simulink library "carnot"  (R2013b)
settings: Solver=ode45  StartTime=0.0  StopTime=10.0  RelTol=1e-3
undefined symbols (not defined in the file or in its folder): A, acol, Ahabit, Awin, Azimuth_Angle, AziWin, B, C, c1, c4, capc, caph, CarnotCallbacks_Density, CarnotCallbacks_Enthalpy, CarnotCallbacks_Enthalpy2Temperature, CarnotCallbacks_Entropy, CarnotCallbacks_Evaporation_Enthalpy, CarnotCallbacks_GlobalMessageLevel, CarnotCallbacks_Grashof, CarnotCallbacks_Heat_Capacity, CarnotCallbacks_Kinematic_Viscosity, CarnotCallbacks_Prandtl, CarnotCallbacks_Saturation_Property, CarnotCallbacks_Saturation_Temperature, CarnotCallbacks_Saturation_Value_Water, CarnotCallbacks_Specific_Volume, CarnotCallbacks_Thermal_Conductivity, CarnotCallbacks_Vapour_Content, CarnotCallbacks_Vapour_Pressure, con, cond, d, Dd, density, dfin, dia, DiameterLastPiece, DPConstant, dpipe, DPLinear, DPQuadratic, emission_out, fluid, FluidMix, FluidType, FPC, frame, g, GeodeticHeight, Gwin, heat_capacity, hgt, HP, Hroom, ID, inlet, K, l, lin, lpipe ... (+29)
undefined symbols (not defined in the file): c2, c3, c5, c6, cwall, dactive, height, mc, mID, rho, tau, UAneighbour, UAwall, uloss
libraries: carnot x333, simulink x25, simulink_extras x7
(part 4 of 16)

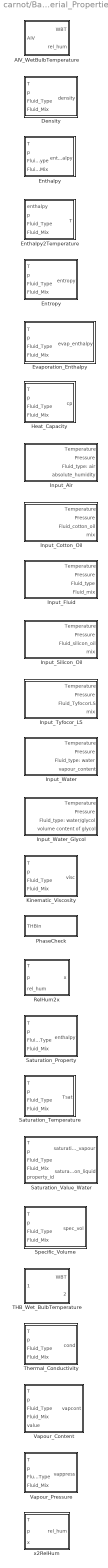
== system carnot/Basic/Material_Properties ==
  AIV_WetBulbTemperature : Subsystem  mask(AIV to wet bulb temperature and relative humidity){}
      mask help:
      | Calculate  - the relative humidity of air (rH)
      |                  - and the wet bulb temperature of air (WBT)
      | from          - dry bulb air temperature (DBT)
      |                  - and mass of water per mass of air (x)
      | in AIV vector.
      |
      | DBT        [degree centigrade]
      | p              [Pa]
      | x              kg water / kg air
      |
      | rel_hum   [percent]
      | WBT       [degree centigrade] -> T_WBT is valid for T [-6..40°C]
      mask Help: web(fullfile(path_carnot('help'),'wetbulbtemperature.html'),'-helpbrowser')
  Density : Subsystem  LoadFcn=CarnotCallbacks_Density('LoadFcn');  InitFcn=load('THB.mat');  VariantControl=CarlibClassic  mask(density){INPUTARGUMENTS=state variables (classic), DEBUGLEVEL=DEBUGLEVEL, MAXTOTALWARNINGS=inf, MAXCONSECUTIVEWARNINGS=inf, WRITETOFILE=0, FILENAME='errors.txt'}
      mask prompts: INPUTARGUMENTS "Input arguments"; DEBUGLEVEL "Debug level"; MAXTOTALWARNINGS "maximum number of total warning"; MAXCONSECUTIVEWARNINGS "maximum number of consecutive warnings"; WRITETOFILE "write messages to file"; FILENAME "filename for error messages"
      mask help:
      | Calculates the fluid density  [kg/m³]. Calls the function "density" in the CARNOT library "carlib".
      | You may use the block "GlobalMessageLevel" in the Toolbox to handle the debugging messages.
      | FluidType        Remarks
      | 1: water          fluid mix is vapourcontent in the 2-phase region
      | 2: air              fluid mix is (kg water) / (kg dry air)
      | 3: cotton oil       -
      | 4: silicone oil     -
      | 5: water-glycol   fluid mix is volume partition [0..1] of propylen glycol
      | 6: Tyfocor LS     function only available in liquid phase
      | 7: Water Constant = 998.21 kg/m³ (water at 20°C)
      | 8: Air Constant   = 1.118 kg/m³ (air at 20°C)
      mask init:
      | %Inports
      | CarnotCallbacks_Density('CreateInports');
      | 
      | %global debug level
      | [DEBUGLEVEL, MAXTOTALWARNINGS, MAXCONSECUTIVEWARNINGS, WRITETOFILE, FILENAME] = CarnotCallbacks_Density('CheckDebugLevels', DEBUGLEVEL, MAXTOTALWARNINGS, MAXCONSECUTIVEWARNINGS, WRITETOFILE, FILENAME);
      mask Help: web(fullfile(path_carnot('help'),'density.html'),'-helpbrowser')
      mask TypeOptions INPUTARGUMENTS: state variables (classic) | THB | THV
      mask Callback INPUTARGUMENTS: CarnotCallbacks_Density('MaskVisibilities');
      mask TypeOptions DEBUGLEVEL: DEBUGLEVEL | INFOLEVEL | WARNINGLEVEL | ERRORLEVEL | FATALLEVEL | NOLEVEL
  Enthalpy : Subsystem  LoadFcn=CarnotCallbacks_Enthalpy('LoadFcn');  InitFcn=load('THB.mat');  VariantControl=CarlibClassic  mask(enthalpy){INPUTARGUMENTS=state variables (classic), DEBUGLEVEL=WARNINGLEVEL, MAXTOTALMESSAGES=inf, MAXCONSECUTIVEMESSAGES=inf, WRITETOFILE=0, FILENAME='errors.txt'}
      mask prompts: INPUTARGUMENTS "Input arguments"; DEBUGLEVEL "Debug level"; MAXTOTALMESSAGES "maximum number of total warning"; MAXCONSECUTIVEMESSAGES "maximum number of consecutive warnings"; WRITETOFILE "write messages to file"; FILENAME "filename for error messages"
      mask help:
      | Calculates the fluid specific enthalpy  [J/kg].
      | Calls the CARNOT library "carlib".
      | WORKS FOR WATER AND DRY AIR! Enthalpy for other fluids is cp*T.
      | FluidType        Remarks
      | 1: water          fluid mix is vapourcontent in the 2-phase region
      | 2: air              fluid mix is (kg water) / (kg dry air)
      | 3: cotton oil       -
      | 4: silicone oil     -
      | 5: water-glycol   fluid mix is volume partition [0..1] of propylen glycol
      | 6: Tyfocor LS     function only available in liquid phase
      | 7: Water Constant = 0.0 J/kg (water at 20°C)
      | 8: Air Constant   = 0.0 J/kg (air at 20°C)
      mask init:
      | %Inports
      | CarnotCallbacks_Enthalpy('CreateInports');
      | 
      | %global debug level
      | [DEBUGLEVEL, MAXTOTALMESSAGES, MAXCONSECUTIVEMESSAGES, WRITETOFILE, FILENAME] = CarnotCallbacks_Enthalpy('CheckDebugLevels', DEBUGLEVEL, MAXTOTALMESSAGES, MAXCONSECUTIVEMESSAGES, WRITETOFILE, FILENAME);
      mask Help: web(fullfile(path_carnot('help'),'enthalpy.html'),'-helpbrowser')
      mask TypeOptions INPUTARGUMENTS: state variables (classic) | THB | THV
      mask Callback INPUTARGUMENTS: CarnotCallbacks_Enthalpy('MaskVisibilities');
      mask TypeOptions DEBUGLEVEL: DEBUGLEVEL | INFOLEVEL | WARNINGLEVEL | ERRORLEVEL | FATALLEVEL | NOLEVEL
  Enthalpy2Temperature : Subsystem  LoadFcn=CarnotCallbacks_Enthalpy2Temperature('LoadFcn');  VariantControl=CarlibClassic  mask(Enthalpy to Temperature){DEBUGLEVEL=WARNINGLEVEL, MAXTOTALMESSAGES=inf, MAXCONSECUTIVEMESSAGES=inf, WRITETOFILE=0, FILENAME='errors.txt'}
      mask prompts: DEBUGLEVEL "Debug level"; MAXTOTALMESSAGES "maximum number of total warning"; MAXCONSECUTIVEMESSAGES "maximum number of consecutive warnings"; WRITETOFILE "write messages to file"; FILENAME "filename for error messages"
      mask help:
      | Calculates the temperature  [°C] from the fluid Enthalpy [J/kg].
      | Enthalpy may be a scalar or a vector. All other inputs must be scalar.
      | FluidType        Remarks
      | 1: water          fluid mix is vapourcontent in the 2-phase region
      | 2: air              fluid mix is (kg water) / (kg dry air)
      | 3: cotton oil       -
      | 4: silicone oil     -
      | 5: water-glycol   fluid mix is volume partition [0..1] of propylen glycol
      | 6: Tyfocor LS     function only available in liquid phase
      | 7: Water Constant - function not defined
      | 8: Air Constant - function not defined
      mask init:
      | %global debug level
      | [DEBUGLEVEL, MAXTOTALMESSAGES, MAXCONSECUTIVEMESSAGES, WRITETOFILE, FILENAME] = CarnotCallbacks_Enthalpy2Temperature('CheckDebugLevels', DEBUGLEVEL, MAXTOTALMESSAGES, MAXCONSECUTIVEMESSAGES, WRITETOFILE, FILENAME);
      mask Help: web(fullfile(path_carnot('help'),'enthalpy2temperature.html'),'-helpbrowser')
      mask TypeOptions DEBUGLEVEL: DEBUGLEVEL | INFOLEVEL | WARNINGLEVEL | ERRORLEVEL | FATALLEVEL | NOLEVEL
      mask DialogControl ParameterTabVar0 Prompt: Debugging
  Entropy : Subsystem  LoadFcn=CarnotCallbacks_Entropy('LoadFcn');  InitFcn=load('THB.mat');  VariantControl=CarlibClassic  mask(entropy){INPUTARGUMENTS=state variables (classic), DEBUGLEVEL=WARNINGLEVEL, MAXTOTALMESSAGES=inf, MAXCONSECUTIVEMESSAGES=inf, WRITETOFILE=0, FILENAME='errors.txt'}
      mask prompts: INPUTARGUMENTS "Input arguments"; DEBUGLEVEL "Debug level"; MAXTOTALMESSAGES "maximum number of total warning"; MAXCONSECUTIVEMESSAGES "maximum number of consecutive warnings"; WRITETOFILE "write messages to file"; FILENAME "filename for error messages"
      mask help:
      | The block calculates the entropy  [J/kgK] of the fluid.
      | The block calls the function "entropy" in the CARNOT library "carlib".
      | FluidType        Remarks
      | 1: water          fluid mix is vapourcontent in the 2-phase region
      | 2: air              fluid mix is (kg water) / (kg dry air)
      | 3: cotton oil       -
      | 4: silicone oil     -
      | 5: water-glycol   fluid mix is volume partition [0..1] of propylen glycol
      | 6: Tyfocor LS     function only available in liquid phase
      | 7: Water Constant = 0.0 J/K/kg
      | 8: Air Constant   = 0.0 J/K/kg
      mask init:
      | %Inports
      | CarnotCallbacks_Entropy('CreateInports');
      | 
      | %global debug level
      | [DEBUGLEVEL, MAXTOTALMESSAGES, MAXCONSECUTIVEMESSAGES, WRITETOFILE, FILENAME] = CarnotCallbacks_Entropy('CheckDebugLevels', DEBUGLEVEL, MAXTOTALMESSAGES, MAXCONSECUTIVEMESSAGES, WRITETOFILE, FILENAME);
      mask Help: web(fullfile(path_carnot('help'),'entropy.html'),'-helpbrowser')
      mask TypeOptions INPUTARGUMENTS: state variables (classic) | THB | THV
      mask Callback INPUTARGUMENTS: CarnotCallbacks_Entropy('MaskVisibilities');
      mask TypeOptions DEBUGLEVEL: DEBUGLEVEL | INFOLEVEL | WARNINGLEVEL | ERRORLEVEL | FATALLEVEL | NOLEVEL
  Evaporation_Enthalpy : Subsystem  LoadFcn=CarnotCallbacks_Evaporation_Enthalpy('LoadFcn');  InitFcn=load('THB.mat');  VariantControl=CarlibClassic  mask(entropy){INPUTARGUMENTS=state variables (classic), DEBUGLEVEL=WARNINGLEVEL, MAXTOTALMESSAGES=inf, MAXCONSECUTIVEMESSAGES=inf, WRITETOFILE=0, FILENAME='errors.txt'}
      mask prompts: INPUTARGUMENTS "Input arguments"; DEBUGLEVEL "Debug level"; MAXTOTALMESSAGES "maximum number of total warning"; MAXCONSECUTIVEMESSAGES "maximum number of consecutive warnings"; WRITETOFILE "write messages to file"; FILENAME "filename for error messages"
      mask help:
      | The block calculates the evaporation enthalpy [J/kgK] of water.
      | The block uses the material properties functions in carlib.
      | FluidType  material           remarks on fluid mix
      | 1           water              vapourcontent in the 2-phase region
      | all others: function not defined
      mask init:
      | %Inports
      | CarnotCallbacks_Evaporation_Enthalpy('CreateInports');
      | 
      | %global debug level
      | [DEBUGLEVEL, MAXTOTALMESSAGES, MAXCONSECUTIVEMESSAGES, WRITETOFILE, FILENAME] = CarnotCallbacks_Evaporation_Enthalpy('CheckDebugLevels', DEBUGLEVEL, MAXTOTALMESSAGES, MAXCONSECUTIVEMESSAGES, WRITETOFILE, FILENAME);
      mask Help: web(fullfile(path_carnot('help'),'evaporation_enthalpy.html'),'-helpbrowser')
      mask TypeOptions INPUTARGUMENTS: state variables (classic) | THB | THV
      mask Callback INPUTARGUMENTS: CarnotCallbacks_Evaporation_Enthalpy('MaskVisibilities');
      mask TypeOptions DEBUGLEVEL: DEBUGLEVEL | INFOLEVEL | WARNINGLEVEL | ERRORLEVEL | FATALLEVEL | NOLEVEL
  Heat_Capacity : Subsystem  LoadFcn=CarnotCallbacks_Heat_Capacity('LoadFcn');  InitFcn=load('THB.mat');  VariantControl=CarlibClassic  mask(heat capacity){INPUTARGUMENTS=state variables (classic), DEBUGLEVEL=DEBUGLEVEL, MAXTOTALWARNINGS=inf, MAXCONSECUTIVEWARNINGS=inf, WRITETOFILE=0, FILENAME='errors.txt'}
      mask prompts: INPUTARGUMENTS "Input arguments"; DEBUGLEVEL "Debug level"; MAXTOTALWARNINGS "maximum number of total warning"; MAXCONSECUTIVEWARNINGS "maximum number of consecutive warnings"; WRITETOFILE "write messages to file"; FILENAME "filename for error messages"
      mask help:
      | Calculates the  heat_capacity of fluids [J/(kg*K)]. Calls calls the function "heat_capacity" in the CARNOT library "carlib".
      | You may use the block "GlobalMessageLevel" in the Toolbox to handle the debugging messages.
      | FluidType        Remarks
      | 1: water          fluid mix is vapourcontent in the 2-phase region
      | 2: air              fluid mix is (kg water) / (kg dry air)
      | 3: cotton oil       -
      | 4: silicone oil     -
      | 5: water-glycol   fluid mix is volume partition [0..1] of propylen glycol
      | 6: Tyfocor LS     function only available in liquid phase
      | 7: Water Constant = 4181.0 J/kg/K (water at 20°C)
      | 8: Air Constant   = 1007.0 J/kg/K (air at 20°C)
      mask init:
      | %Inports
      | CarnotCallbacks_Heat_Capacity('CreateInports');
      | 
      | %global debug level
      | [DEBUGLEVEL, MAXTOTALWARNINGS, MAXCONSECUTIVEWARNINGS, WRITETOFILE, FILENAME] = CarnotCallbacks_Heat_Capacity('CheckDebugLevels', DEBUGLEVEL, MAXTOTALWARNINGS, MAXCONSECUTIVEWARNINGS, WRITETOFILE, FILENAME);
      mask Help: web(fullfile(path_carnot('help'),'heat_capacity.html'),'-helpbrowser')
      mask TypeOptions INPUTARGUMENTS: state variables (classic) | THB | THV
      mask Callback INPUTARGUMENTS: CarnotCallbacks_Heat_Capacity('MaskVisibilities');
      mask TypeOptions DEBUGLEVEL: DEBUGLEVEL | INFOLEVEL | WARNINGLEVEL | ERRORLEVEL | FATALLEVEL | NOLEVEL
  Input_Air : Subsystem  mask(Input_Air){T=20, p=1e5, x=0.005}
      mask prompts: T "temperature (scalar or vector) [°C]"; p "pressure [Pa]"; x "absolute humidity of moist air [kg water/kg dry air]"
      mask help:
      | Input block for the material "Air"
      |
      | The relevant inputs for the calculation of the block can be specified as parameter in the mask
      mask Help: web(fullfile(path_carnot('help'),'input_material.html'),'-helpbrowser')
  Input_Cotton_Oil : Subsystem  mask(Input_Cotton_Oil){T=20, p=1e5}
      mask prompts: T "temperature (scalar or vector) [°C]"; p "pressure [Pa]"
      mask help: Input block for the material "Cotton Oil". The relevant inputs for the calculation of the block can be specified as parameter in the mask
      mask Help: web(fullfile(path_carnot('help'),'input_material.html'),'-helpbrowser')
  Input_Fluid : Subsystem  mask(Input_Fluid){fluid=Water, T=[10:10:50], p=1e5, x=0.005}
      mask prompts: fluid "Fluid type"; T "temperature (scalar or vector) [°C]"; p "pressure [Pa]"; x "Fluid Mix"
      mask help:
      | FLUID            FLUID MIX
      | water          vapourcontent in the 2-phase region
      | air               (kg water) / (kg dry air)
      | cotton oil       -
      | silicone oil     -
      | water-glycol   volume partition [0..1] of propylen glycol
      mask Help: web(fullfile(path_carnot('help'),'input_material.html'),'-helpbrowser')
      mask TypeOptions fluid: Water | Air | Cotton Oil | Silicone Oil | Water-Glycol Mix | Tyfocor LS | Water (Constant 20°C) | Air (dry+ constant 20°C)
  Input_Silicon_Oil : Subsystem  mask(Input_Silicon_Oil){T=20, p=1e5}
      mask prompts: T "temperature (scalar or vector) [°C]"; p "pressure [Pa]"
      mask help: Input block for the material "Silicon_Oil". The relevant inputs for the calculation of the block can be specified as parameter in the mask
      mask Help: web(fullfile(path_carnot('help'),'input_material.html'),'-helpbrowser')
  Input_Tyfocor_LS : Subsystem  mask(Input_Tyfocor_LS){T=20, p=1e5}
      mask prompts: T "temperature (scalar or vector) [°C]"; p "pressure [Pa]"
      mask help:
      | Input block for the material "Tyfocor_LS". The relevant inputs for the calculation of the block can be specified as parameter in the mask.
      | Tyfocor is a registered trademark of Tyforop Chemie, Hamburg (Germany).
      mask Help: web(fullfile(path_carnot('help'),'input_material.html'),'-helpbrowser')
  Input_Water : Subsystem  mask(Input_Water){T=20, p=2e6, xd=0}
      mask prompts: T "temperature (scalar or vector) [°C]"; p "pressure [Pa]"; xd "vapour content of the water [0..1]"
      mask help:
      | Input block for the material "Water"
      |
      | The relevant inputs for the calculation of the block can be specified as parameter in the mask
      mask Help: web(fullfile(path_carnot('help'),'input_material.html'),'-helpbrowser')
  Input_Water_Glycol : Subsystem  mask(input_water_glycol){T=20, p=1e5, g=0.4}
      mask prompts: T "temperature (scalar or vector) [°C]"; p "pressure [Pa]"; g "volume content of glycol [0..1]"
      mask help: Sets all values for the water - propylen-glycol mixtures.
      mask Help: web(fullfile(path_carnot('help'),'input_material.html'),'-helpbrowser')
  Kinematic_Viscosity : Subsystem  LoadFcn=CarnotCallbacks_Kinematic_Viscosity('LoadFcn');  InitFcn=load('THB.mat');  VariantControl=CarlibClassic  mask(kinematic viscosity){INPUTARGUMENTS=state variables (classic), DEBUGLEVEL=WARNINGLEVEL, MAXTOTALMESSAGES=inf, MAXCONSECUTIVEMESSAGES=inf, WRITETOFILE=0, FILENAME='errors.txt'}
      mask prompts: INPUTARGUMENTS "Input arguments"; DEBUGLEVEL "Debug level"; MAXTOTALMESSAGES "maximum number of total warning"; MAXCONSECUTIVEMESSAGES "maximum number of consecutive warnings"; WRITETOFILE "write messages to file"; FILENAME "filename for error messages"
      mask help:
      | Calculates the kinematic viscosity of fluids [m²/s].
      | Calls the function "viscosity" in the CARNOT library "carlib".
      | FluidType        Remarks
      | 1: water          fluid mix is vapourcontent in the 2-phase region
      | 2: air              fluid mix is (kg water) / (kg dry air)
      | 3: cotton oil       -
      | 4: silicone oil     -
      | 5: water-glycol   fluid mix is volume partition [0..1] of propylen glycol
      | 6: Tyfocor LS     function only available in liquid phase
      | 7: Water Constant = 1.004e-6 m²/s (water at 20°C)
      | 8: Air Constant   = 15.35e-6 m²/s (air at 20°C)
      mask init:
      | %Inports
      | CarnotCallbacks_Kinematic_Viscosity('CreateInports');
      | 
      | %global debug level
      | [DEBUGLEVEL, MAXTOTALMESSAGES, MAXCONSECUTIVEMESSAGES, WRITETOFILE, FILENAME] = CarnotCallbacks_Kinematic_Viscosity('CheckDebugLevels', DEBUGLEVEL, MAXTOTALMESSAGES, MAXCONSECUTIVEMESSAGES, WRITETOFILE, FILENAME);
      mask Help: web(fullfile(path_carnot('help'),'kinematic_viscosity.html'),'-helpbrowser')
      mask TypeOptions INPUTARGUMENTS: state variables (classic) | THB | THV
      mask Callback INPUTARGUMENTS: CarnotCallbacks_Kinematic_Viscosity('MaskVisibilities');
      mask TypeOptions DEBUGLEVEL: DEBUGLEVEL | INFOLEVEL | WARNINGLEVEL | ERRORLEVEL | FATALLEVEL | NOLEVEL
  PhaseCheck : Subsystem  mask(phasecheck){}
      mask help: Checks whether fluid is still in the correct phase, for example if water is not steam or ice. Simulation is stopped for inconstistent phase.
      mask Help: web(fullfile(path_carnot('help'),'phase_check.html'),'-helpbrowser')
  RelHum2x : Subsystem  mask(relative humidity to x){}
      mask help:
      | Calculate the mass of water per mass of air (x)
      | from the relative humidity of air.
      |
      | T             [degree centigrade]
      | p             [Pa]
      | rel_hum   [percent]
      | x              kg water / kg air
      mask Help: web(fullfile(path_carnot('help'),'rel_hum2x.html'),'-helpbrowser')
  Saturation_Property : Subsystem  LoadFcn=CarnotCallbacks_Saturation_Property('LoadFcn');  InitFcn=load('THB.mat');  VariantControl=CarlibClassic  mask(saturation property){INPUTARGUMENTS=state variables (classic), PROPERTY=density, FLUIDPHASE=liquid, DEBUGLEVEL=WARNINGLEVEL, MAXTOTALMESSAGES=inf, MAXCONSECUTIVEMESSAGES=inf, WRITETOFILE=0, FILENAME='errors.txt'}
      mask prompts: INPUTARGUMENTS "Input arguments"; FLUIDPHASE "fluid phase"; DEBUGLEVEL "Debug level"; MAXTOTALMESSAGES "maximum number of total warning"; MAXCONSECUTIVEMESSAGES "maximum number of consecutive warnings"; WRITETOFILE "write messages to file"; FILENAME "filename for error messages"
      mask help:
      | The block calculates the saturation value of water by the value of a specified property. Calls the function "saturationproperty" in the CARNOT library "Carlib".
      |
      | PROPERTY            UNIT
      | density                     kg/m³
      | heat capacity           J/kgK
      | heat conductivity     W/mK
      | kinematic viscosity   m²/s
      | enthalpy                   J/kg
      | entropy                     J/kgK
      | prandtl                      --
      | specific volume        m³/kg
      mask init:
      | %Inports
      | CarnotCallbacks_Saturation_Property('CreateInports');
      | 
      | %global debug level
      | [DEBUGLEVEL, MAXTOTALMESSAGES, MAXCONSECUTIVEMESSAGES, WRITETOFILE, FILENAME] = CarnotCallbacks_Saturation_Property('CheckDebugLevels', DEBUGLEVEL, MAXTOTALMESSAGES, MAXCONSECUTIVEMESSAGES, WRITETOFILE, FILENAME);
      mask Help: web(fullfile(path_carnot('help'),'saturationproperty.html'),'-helpbrowser')
      mask TypeOptions INPUTARGUMENTS: state variables (classic) | THB | THV
      mask Callback INPUTARGUMENTS: CarnotCallbacks_Saturation_Property('MaskVisibilities');
      mask TypeOptions PROPERTY: density | heat capacity | heat conductivity | kinematic viscosity | enthalpy | entropy | prandtl | specific volume
      mask TypeOptions FLUIDPHASE: vaporous | liquid | solid
      mask TypeOptions DEBUGLEVEL: DEBUGLEVEL | INFOLEVEL | WARNINGLEVEL | ERRORLEVEL | FATALLEVEL | NOLEVEL
  Saturation_Temperature : Subsystem  LoadFcn=CarnotCallbacks_Saturation_Temperature('LoadFcn');  InitFcn=load('THB.mat');  VariantControl=CarlibClassic  mask(Saturation Temperature){INPUTARGUMENTS=state variables (classic), DEBUGLEVEL=WARNINGLEVEL, MAXTOTALMESSAGES=inf, MAXCONSECUTIVEMESSAGES=inf, WRITETOFILE=0, FILENAME='errors.txt'}
      mask prompts: INPUTARGUMENTS "Input arguments"; DEBUGLEVEL "Debug level"; MAXTOTALMESSAGES "maximum number of total warning"; MAXCONSECUTIVEMESSAGES "maximum number of consecutive warnings"; WRITETOFILE "write messages to file"; FILENAME "filename for error messages"
      mask help:
      | Calculates the saturationtemperature in °C
      | Fluid Type 1 - water or water mixtures: temperature of saturated steam as a function of pressure.
      | Fluid Type 2 - moist air: dew point temperature of the moist air as a function of water content. Input fluid mix (kg water / kg air) may be a vector.
      mask init:
      | %Inports
      | CarnotCallbacks_Saturation_Temperature('CreateInports');
      | 
      | %global debug level
      | [DEBUGLEVEL, MAXTOTALMESSAGES, MAXCONSECUTIVEMESSAGES, WRITETOFILE, FILENAME] = CarnotCallbacks_Saturation_Temperature('CheckDebugLevels', DEBUGLEVEL, MAXTOTALMESSAGES, MAXCONSECUTIVEMESSAGES, WRITETOFILE, FILENAME);
      mask Help: web(fullfile(path_carnot('help'),'saturation_temperature.html'),'-helpbrowser')
      mask TypeOptions INPUTARGUMENTS: state variables (classic) | THB | THV
      mask Callback INPUTARGUMENTS: CarnotCallbacks_Saturation_Temperature('MaskVisibilities');
      mask TypeOptions DEBUGLEVEL: DEBUGLEVEL | INFOLEVEL | WARNINGLEVEL | ERRORLEVEL | FATALLEVEL | NOLEVEL
  Saturation_Value_Water : Subsystem  LoadFcn=CarnotCallbacks_Saturation_Value_Water('LoadFcn');  InitFcn=load('THB.mat');  VariantControl=CarlibClassic  mask(saturation value water){INPUTARGUMENTS=state variables (classic), DEBUGLEVEL=WARNINGLEVEL, MAXTOTALMESSAGES=inf, MAXCONSECUTIVEMESSAGES=inf, WRITETOFILE=0, FILENAME='errors.txt'}
      mask prompts: INPUTARGUMENTS "Input arguments"; DEBUGLEVEL "Debug level"; MAXTOTALMESSAGES "maximum number of total warning"; MAXCONSECUTIVEMESSAGES "maximum number of consecutive warnings"; WRITETOFILE "write messages to file"; FILENAME "filename for error messages"
      mask help:
      | Calculates the saturation value of fluid by the value of a specified property.
      | Temperature may be a scalar or vector, all other inputs must be scalar.
      | property-ID        property                       unit
      | 1                       density                         [kg/m³]
      | 2                       heat capacity               [J/kgK]
      | 3                       heat conductivity         [W/mK]
      | 4                       kinematic viscosity       [m²/s]
      | 5                       enthalpy                       [J/kg]
      | 6                       entropy                         [J/kgK]
      | 7                       prandtl                          [-]
      | 8                       specific volume            [m³/kg]
      | not defined for this function
      | 9                       evaporation  enthalpy  [J/kg]
      | 10                     vapourpressure            [Pa]
      | 11                     saturationtemperatur    [°C]
      mask init:
      | %Inports
      | CarnotCallbacks_Saturation_Value_Water('CreateInports');
      | 
      | %global debug level
      | [DEBUGLEVEL, MAXTOTALMESSAGES, MAXCONSECUTIVEMESSAGES, WRITETOFILE, FILENAME] = CarnotCallbacks_Saturation_Value_Water('CheckDebugLevels', DEBUGLEVEL, MAXTOTALMESSAGES, MAXCONSECUTIVEMESSAGES, WRITETOFILE, FILENAME);
      mask Help: web(fullfile(path_carnot('help'),'saturationvalue_water.html'),'-helpbrowser')
      mask TypeOptions INPUTARGUMENTS: state variables (classic) | THB | THV
      mask Callback INPUTARGUMENTS: CarnotCallbacks_Saturation_Value_Water('MaskVisibilities');
      mask TypeOptions DEBUGLEVEL: DEBUGLEVEL | INFOLEVEL | WARNINGLEVEL | ERRORLEVEL | FATALLEVEL | NOLEVEL
  Specific_Volume : Subsystem  LoadFcn=CarnotCallbacks_Specific_Volume('LoadFcn');  InitFcn=load('THB.mat');  VariantControl=CarlibClassic  mask(specific volume){INPUTARGUMENTS=state variables (classic), DEBUGLEVEL=DEBUGLEVEL, MAXTOTALWARNINGS=inf, MAXCONSECUTIVEWARNINGS=inf, WRITETOFILE=0, FILENAME='errors.txt'}
      mask prompts: INPUTARGUMENTS "Input arguments"; DEBUGLEVEL "Debug level"; MAXTOTALWARNINGS "maximum number of total warning"; MAXCONSECUTIVEWARNINGS "maximum number of consecutive warnings"; WRITETOFILE "write messages to file"; FILENAME "filename for error messages"
      mask help:
      | Calculates the specific volume of fluids [m³/kg]. Calls the function "specific_volume" in the CARNOT library "Carlib".
      | You may use the block "GlobalMessageLevel" in the Toolbox to handle the debugging messages.
      | FluidType        Remarks
      | 1: water          fluid mix is vapourcontent in the 2-phase region
      | 2: air              fluid mix is (kg water) / (kg dry air)
      | 3: cotton oil       -
      | 4: silicone oil     -
      | 5: water-glycol   fluid mix is volume partition [0..1] of propylen glycol
      | 6: Tyfocor LS     function only available in liquid phase
      | 7: Water Constant = 1.0 / 998.21 m³/kg (water at 20°C)
      | 8: Air Constant   = 1.0 / 1.118 m³/kg (air at 20°C)
      mask init:
      | %Inports
      | CarnotCallbacks_Specific_Volume('CreateInports');
      | 
      | %global debug level
      | [DEBUGLEVEL, MAXTOTALWARNINGS, MAXCONSECUTIVEWARNINGS, WRITETOFILE, FILENAME] = CarnotCallbacks_Specific_Volume('CheckDebugLevels', DEBUGLEVEL, MAXTOTALWARNINGS, MAXCONSECUTIVEWARNINGS, WRITETOFILE, FILENAME);
      mask Help: web(fullfile(path_carnot('help'),'specific_volume.html'),'-helpbrowser')
      mask TypeOptions INPUTARGUMENTS: state variables (classic) | THB | THV
      mask Callback INPUTARGUMENTS: CarnotCallbacks_Specific_Volume('MaskVisibilities');
      mask TypeOptions DEBUGLEVEL: DEBUGLEVEL | INFOLEVEL | WARNINGLEVEL | ERRORLEVEL | FATALLEVEL | NOLEVEL
  THB_Wet_BulbTemperature : Subsystem  mask(THB to wet bulb temperature and relative humidity){}
      mask help:
      | Calculate  - the relative humidity of air (rH)
      |                  - and the wet bulb temperature of air (WBT)
      | from          - dry bulb air temperature (DBT)
      |                  - and mass of water per mass of air (x)
      | in THV vector.
      |
      | DBT        [degree centigrade]
      | p              [Pa]
      | x              kg water / kg air
      |
      | rel_hum   [percent]
      | WBT       [degree centigrade] -> T_WBT is valid for T [-6..40°C]
      mask Help: web(fullfile(path_carnot('help'),'wetbulbtemperature.html'),'-helpbrowser')
  Thermal_Conductivity : Subsystem  LoadFcn=CarnotCallbacks_Thermal_Conductivity('LoadFcn');  InitFcn=load('THB.mat');  VariantControl=CarlibClassic  mask(thermal conductivity){INPUTARGUMENTS=state variables (classic), DEBUGLEVEL=WARNINGLEVEL, MAXTOTALMESSAGES=inf, MAXCONSECUTIVEMESSAGES=inf, WRITETOFILE=0, FILENAME='errors.txt'}
      mask prompts: INPUTARGUMENTS "Input arguments"; DEBUGLEVEL "Debug level"; MAXTOTALMESSAGES "maximum number of total warning"; MAXCONSECUTIVEMESSAGES "maximum number of consecutive warnings"; WRITETOFILE "write messages to file"; FILENAME "filename for error messages"
      mask help:
      | Calclulates the heat conductivity of fluids in [W/(m*K)]. Calls the function "cond" in the CARNOT library "carlib".
      | Temperature input may be a vector with several elements.
      | You may use the block "GlobalMessageLevel" in the Toolbox to handle the debugging messages.
      | FluidType        Remarks
      | 1: water          fluid mix is vapourcontent in the 2-phase region
      | 2: air              fluid mix is (kg water) / (kg dry air)
      | 3: cotton oil       -
      | 4: silicone oil     -
      | 5: water-glycol   fluid mix is volume partition [0..1] of propylen glycol
      | 6: Tyfocor LS     function only available in liquid phase
      | 7: Water Constant =  0.5984 W/m/K (water at 20°C)
      | 8: Air Constant   =  0.02569 W/m/K (air at 20°C)
      mask init:
      | %Inports
      | CarnotCallbacks_Thermal_Conductivity('CreateInports');
      | 
      | %global debug level
      | [DEBUGLEVEL, MAXTOTALMESSAGES, MAXCONSECUTIVEMESSAGES, WRITETOFILE, FILENAME] = CarnotCallbacks_Thermal_Conductivity('CheckDebugLevels', DEBUGLEVEL, MAXTOTALMESSAGES, MAXCONSECUTIVEMESSAGES, WRITETOFILE, FILENAME);
      mask Help: web(fullfile(path_carnot('help'),'thermal_conductivity.html'),'-helpbrowser')
      mask TypeOptions INPUTARGUMENTS: state variables (classic) | THB | THV
      mask Callback INPUTARGUMENTS: CarnotCallbacks_Thermal_Conductivity('MaskVisibilities');
      mask TypeOptions DEBUGLEVEL: DEBUGLEVEL | INFOLEVEL | WARNINGLEVEL | ERRORLEVEL | FATALLEVEL | NOLEVEL
  Vapour_Content : Subsystem  LoadFcn=CarnotCallbacks_Vapour_Content('LoadFcn');  InitFcn=load('THB.mat');  VariantControl=CarlibClassic  mask(vapourcontent){INPUTARGUMENTS=state variables (classic), PROPERTYTYPE=density, DEBUGLEVEL=WARNINGLEVEL, MAXTOTALMESSAGES=inf, MAXCONSECUTIVEMESSAGES=inf, WRITETOFILE=0, FILENAME='errors.txt'}
      mask prompts: INPUTARGUMENTS "Input arguments"; PROPERTYTYPE "property type"; DEBUGLEVEL "Debug level"; MAXTOTALMESSAGES "maximum number of total warning"; MAXCONSECUTIVEMESSAGES "maximum number of consecutive warnings"; WRITETOFILE "write messages to file"; FILENAME "filename for error messages"
      mask help:
      | The block calculates the (water-)vapour content of water or water-glycol mixture by the value of a specified property. The block calls the function "vapourcontent" in the CARNOT library "Carlib".
      | Temperature and the "Value" may be a scalar or vector, all other inputs must be scalar (length of "temperature" and "value" must be same).
      | You may use the block "GlobalMessageLevel" in the Toolbox to handle the debugging messages.
      | Definition of property-types
      | property                    unit
      |  density                     [kg/m³]
      |  heat capacity           [J/kgK]
      |  heat conductivity     [W/mK]
      |  kinematic viscosity   [m²/s]
      |  enthalpy                   [J/kg]
      |  entropy                     [J/kgK]
      |  prandtl                      [-]
      |  specific volume        [m³/kg]
      mask init:
      | %Inports
      | CarnotCallbacks_Vapour_Content('CreateInports');
      | 
      | %global debug level
      | [DEBUGLEVEL, MAXTOTALMESSAGES, MAXCONSECUTIVEMESSAGES, WRITETOFILE, FILENAME] = CarnotCallbacks_Vapour_Content('CheckDebugLevels', DEBUGLEVEL, MAXTOTALMESSAGES, MAXCONSECUTIVEMESSAGES, WRITETOFILE, FILENAME);
      mask Help: web(fullfile(path_carnot('help'),'vapour_content.html'),'-helpbrowser')
      mask TypeOptions INPUTARGUMENTS: state variables (classic) | THB | THV
      mask Callback INPUTARGUMENTS: CarnotCallbacks_Vapour_Content('MaskVisibilities');
      mask TypeOptions PROPERTYTYPE: density | heat capacity | heat conductivity | kinematic viscosity | enthalpy | entropy | prandtl | specific volume
      mask TypeOptions DEBUGLEVEL: DEBUGLEVEL | INFOLEVEL | WARNINGLEVEL | ERRORLEVEL | FATALLEVEL | NOLEVEL
  Vapour_Pressure : Subsystem  LoadFcn=CarnotCallbacks_Vapour_Pressure('LoadFcn');  InitFcn=load('THB.mat');  VariantControl=CarlibClassic  mask(vapourpressure){INPUTARGUMENTS=state variables (classic), DEBUGLEVEL=WARNINGLEVEL, MAXTOTALMESSAGES=inf, MAXCONSECUTIVEMESSAGES=inf, WRITETOFILE=0, FILENAME='errors.txt'}
      mask prompts: INPUTARGUMENTS "Input arguments"; DEBUGLEVEL "Debug level"; MAXTOTALMESSAGES "maximum number of total warning"; MAXCONSECUTIVEMESSAGES "maximum number of consecutive warnings"; WRITETOFILE "write messages to file"; FILENAME "filename for error messages"
      mask help:
      | Calculates the vapour pressure of fluids [Pa]. Calls the function "vapourpressure" in the CARNOT library "Carlib".
      | You may use the block "GlobalMessageLevel" in the Toolbox to handle the debugging messages.
      | FluidType        Remarks
      | 1: water          fluid mix is vapourcontent in the 2-phase region
      | 2: air              fluid mix is (kg water) / (kg dry air)
      | 3: cotton oil       function not defined
      | 4: silicone oil     function not defined
      | 5: water-glycol   fluid mix is volume partition [0..1] of propylen glycol
      | 6: Tyfocor LS     function only available in liquid phase
      | 7: Water Constant function not defined
      | 8: Air Constant   function not defined
      mask init:
      | %Inports
      | CarnotCallbacks_Vapour_Pressure('CreateInports');
      | 
      | %global debug level
      | [DEBUGLEVEL, MAXTOTALMESSAGES, MAXCONSECUTIVEMESSAGES, WRITETOFILE, FILENAME] = CarnotCallbacks_Vapour_Pressure('CheckDebugLevels', DEBUGLEVEL, MAXTOTALMESSAGES, MAXCONSECUTIVEMESSAGES, WRITETOFILE, FILENAME);
      mask Help: web(fullfile(path_carnot('help'),'vapourpressure.html'),'-helpbrowser')
      mask TypeOptions INPUTARGUMENTS: state variables (classic) | THB | THV
      mask Callback INPUTARGUMENTS: CarnotCallbacks_Vapour_Pressure('MaskVisibilities');
      mask TypeOptions DEBUGLEVEL: DEBUGLEVEL | INFOLEVEL | WARNINGLEVEL | ERRORLEVEL | FATALLEVEL | NOLEVEL
  x2RelHum : Subsystem  mask(x to relative humidity){}
      mask help:
      | Calculate  the relative humidity of air
      | from the mass of water per mass of air (x).
      |
      | T             [°C]
      | p             [Pa]
      | rel_hum   [percent]
      | x              kg water / kg dry air
      mask Help: web(fullfile(path_carnot('help'),'x2rel_hum.html'),'-helpbrowser')

== system carnot/Basic/Pressure_Drop ==
  Pressure_Drop_Collector : Subsystem  mask(Pressure Drop Collector){len=1, lin=10, qua=10}
      mask prompts: len "Length of Collector"; lin "lin: linear pressure drop in Pa/(kg/s)"; qua "qua: quadratic pressure drop in Pa/(kg/s)²"
      mask help:
      | Calculates the pressure drop according to constant values of con, lin and qua:
      | dp_dyn = con + lin*mdot + qua*mdot²
      | Static height is taken in account via the collector inclination, the length and the temperatures:
      | dp_stat = density * grav * height
      | Total pressure is dp = dp_dyn + dpstat
      mask Help: web(fullfile(path_carnot('help'),'Pressure_Drop_Collector.html'),'-helpbrowser')
  Pressure_Drop_Fix : Subsystem  mask(fixed pressure drop){con=con, lin=lin, qua=qua}
      mask prompts: con "c : constant (static) pressure drop in Pa"; lin "l : linear pressure drop Pa/(kg/s)"; qua "q : quadratic pressure drop Pa/(kg/s)²"
      mask help:
      | Constant parameters for pressure drop in a flow.
      | dp = c + l*mdot + q*mdot²
      | Calculation is done for ID > 10000 (dp = f(l, q), c is neglected) and ID > 20000 (dp = f(c,l,q)).
      | Applied directly to the THB bus.
      mask Help: web(fullfile(path_carnot('help'),'Pressure_Drop_Fix.html'),'-helpbrowser')
  Pressure_Drop_PipeTheory : Subsystem  mask(theoretical pressure drop of a pipe){dia=0.02, len=1, rough=0.04, nbend=1}
      mask prompts: dia "Diameter in m"; len "Length of pipe in m"; rough "Roughness of pipe in m"; nbend "Number of 90° bends"
      mask help: Calculates the pressure drop in a pipe according to a theoretical model.
      mask Help: web(fullfile(path_carnot('help'),'Pressure_Drop_PipeTheory.html'),'-helpbrowser')
  Pressure_Drop_StorageHX : Subsystem  mask(Pressure drop of tube heat exchanger in a storage){dia=dia, hgt=hgt}
      mask prompts: dia "Diameter in m"; hgt "height difference inlet-outlet"
      mask help:
      | Calculates the pressure drop in a tube heat exchanger according to:
      | dp = qua*mdot^2 + lin*mdot + density*grav*height
      mask Help: web(fullfile(path_carnot('help'),'Pressure_Drop_StorageHX.html'),'-helpbrowser')
  Pressure_Drop_StoragePipe : Subsystem  mask(Pressure drop pipe connection of a storage){dia=dia, hgt=hgt}
      mask prompts: dia "Diameter in m"; hgt "height difference inlet-outlet"
      mask help:
      | Calculates the pressure drop in a pipe connection to a storage according to:
      | dp = qua*mdot^2 + lin*mdot + density*grav*height
      | The temperature for the density is taken from the storage nodes.
      mask Help: web(fullfile(path_carnot('help'),'Pressure_Drop_StoragePipe.html'),'-helpbrowser')
  Pressure_Drop_changeD : Subsystem  mask(Pressure Drop Change Diameter){dia=dia}
      mask prompts: dia "Diameter in m"
      mask help: Calculates the pressure drop due to a diameter change at the inlet (of a pipe).
      mask Help: web(fullfile(path_carnot('help'),'Pressure_Drop_changeD.html'),'-helpbrowser')
  Pressure_Drop_staticHeight : Subsystem  mask(Pressure Drop static Height){}
      mask help:
      | Pressure drop or increase due to statig height.
      | Calculation is done for ID > 20000 (dp = f(h)).
      | dp = height/Nnodes*grav*density(Tnodes)
      | The length of Tnodes defines the number of temperature nodes.
      | The height is between inlet and outlet. It is divided by the number of nodes Nnodes in the temperature vector "Tnodes".
      | Height is positive for outlet above inlet but pressure decreases.
      mask Help: web(fullfile(path_carnot('help'),'Pressure_Drop_staticHeight.html'),'-helpbrowser')
  Pressuredrop : Subsystem  mask(pressure drop){}
      mask help:
      | Pressure drop according to input values of con, lin and qua:
      | dp = con + lin*mdot + qua*mdot²
      | The coefficients are also added to the correponding THB elements.
      mask Help: web(fullfile(path_carnot('help'),'Pressuredrop.html'),'-helpbrowser')

== system carnot/Basic/Thermal_Models ==
  Combustion_Calculation : Subsystem  TreatAsAtomicUnit=on
  HeatPump_basic : Subsystem  mask(heat pump){K=K, caph=caph, capc=capc, UA=UA}
      mask prompts: K "Parameters K (see also HP_param.m)"; caph "thermal capacity hot loop [J/K]"; capc "thermal capacity cold loop [J/K]"; UA "heat loss coefficient [W/K]"
      mask help:
      | Linearized heat pump model, uses measured data according to EN 14511 as input (Schwamberger, K.: Fortschrittsberichete VDI, Nr. 263, 1991).
      | heating power: Qdot_h = K1*Tcold_in + K2*Thot_out + K3
      | electric power: Pel = K4*Tcold_in + K5*Thot_out + K6
      | source power: Qdot_c = -K7*Tcold_in - K8*Thot_out - K9
      | differential equation: cap*dTh/dt = Qdot + mdot*cp*(T_in-T) + UA*(Tamb-T)
      | with: cap = mass * heat_capactiy
      | See hp_param.m for the parameters K1 to K9.
      mask Help: web(fullfile(path_carnot('help'),'HeatPump_basic.html'),'-helpbrowser')
      mask Display: plot(0,-30,120,130,[30,46,36,46,36,46,30],[40,40,50,60,70,80,80],[70,54,64,54,64,54,64,54,64,54,70],[40,40,44,50,55,60,65,70,75,80,80],[56,45],[95,95],[51,51],[82,95])
  House_OneNodeModel : Subsystem  mask(House One Node Model){Ahabit=Ahabit, Hroom=Hroom, tini=tini, UAout=UAwall, mc=mc, UAin=UAneighbour, dtroom=inf, AziWin=AziWin, Awin=Awin, Uwin=Uwin, Gwin=Gwin}
      mask prompts: Ahabit "living surface in m²"; Hroom "height of rooms in m"; tini "initial temperature"; UAout "heat loss of walls and roof in W/K"; mc "total thermal capacity in J/K"; UAin "heat transfer to neighbour in W/K"; dtroom "LIMITED TEMPERATURE CHANGE in K (standard value = 'inf')"; AziWin "orientation of 4 windows (south 0, east -90,west 90)"; Awin "surface of 4 windows in m² (vector)"; Uwin "heat loss coefficient 4 windows in W/m²/K [vector]"; Gwin "light transmittance 4 windows (0..1) * (1 - frame_part) [vector]"
      mask help:
      | Simple model of 1-node room or house. The differential equation is solved:
      | (m*c)house * dT/dt = solar_gain + internal_gain + heating_power - losses_to_ambient - losses_to_neighbour_room
      | The heating power is generated by a radiator or floor heating system. A usual value for the internal gains is 2.3 W/m².
      | The windows have a shading for solar radiation (standard value is 1):
      | solar gain = Solar_Radiation_on_window * light_transmittance * shading_factor
      | Use "look under mask" to set up the models parameters (initial conditions, surfaces characteristics...).
      |
      | LIMITED TEMPERATURE CHANGE: If you want to calculate idealized heating behaviour. 0 K means that the room temperature is fixed, the power balace is the theoretical heating demand (see example_House_Ideal.mdl).
      mask init:
      | invmc = 1/mc;
      | Gwin = max(0,min(1,Gwin));
      mask Help: web(fullfile(path_carnot('help'),'Simple_House.html'),'-helpbrowser')
      mask Display: plot(0,-15,80,100,[30,30,60,60,30],[20,50,50,20,20],[47,47,56,56,47],[40,30,30,40,40],[42,42,34,34],[20,40,40,20],[62,45,28],[48,70,48])
  Pipe_basic : Subsystem  mask(Pipe basic){vol=pi*(d/2)^2*l, L=l, uloss=uloss, effcond=cond, cwall=cwall, t0=t0, nodes=nodes}
      mask prompts: vol "Volume [m³]"; L "Length of pipe [m]"; uloss "Heat loss per pipe length [W/(m*K)]"; effcond "Effective conductivity of pipe wall [W/(m*K)]"; cwall "Capacity of pipewall per length [J/(m*K)]"; t0 "initial temperature [degree centigrade]"; nodes "number of nodes"
      mask help:
      | Multinode pipe with capacity. The flow is calculated by the upwind scheme heat conduction between nodes by central differences (Patankar 1980).
      | heat loss: u = conductivity / ( d_in * ln (d_out / d_in) )
      mask init:
      | nodes = max(nodes, 1);
      | vnode = max(vol,0.0001)/nodes;
      | lnode = max(L, 0.001)/nodes;
      | cnode = max(0.001,cwall)*L/vnode;
      | unode = uloss*lnode/vnode;
      | cond = effcond/(lnode*lnode);
      mask Help: web(fullfile(path_carnot('help'),'Pipe_basic.html'),'-helpbrowser')
      mask Display: plot(0,0,100,100,[24,27,27,24,75,80,80,75,24,20,20,24],[60,53,46,40,40,46,55,60,60,53,46,40])
  Radiator_basic : Subsystem  mask(basic Radiator){pnomEN=1000, dtnomEN=50, expo=1.5, mcp=10*4200}
      mask prompts: pnomEN "Qdot_nom: nominal power in W"; dtnomEN "Tdiff_nom: nominal temperature difference in K"; expo "radiator exponent (> 0)"; mcp "mass * capacity per unit in J/K"
      mask help:
      | The block calculates the heat transfer of a radiator to a room according to the EN 442 equation.
      | Qdot = Qdot_nom * (Tdiff/Tdiff_nom)^n
      mask init:
      | mcap = max(1,mcp); % lower limit for capacity is 1 J/K
      | 
      | % correct values because current model 
      | % uses outlet temperature as mean temperature
      | pnom = pnomEN;
      | dtnom = dtnomEN-5;
      mask Help: web(['file:///' fullfile(path_carnot('help'),'Radiator.html')],'-helpbrowser')
  Solar_Collector_basic : Subsystem  mask(Basic Solar Thermal Collector){acol=acol, c1=c1, c2=c2, c3=c3, c4=c4, c5=c5, c6=c6, tini=tini}
      mask prompts: acol "A : collector surface  [m²]"; c1 "c1 : heat loss coefficient at (Tm-Ta)=0  [W/(m²*K)]"; c2 "c2: temperature dependence of the heat loss coefficient [W/(m*K)²]"; c3 "c3 : wind speed dependence of the heat loss coefficient [J/(m³K)]"; c4 "c4 : sky temperature dependence of the heat loss coefficient [W/(m²K)]"; c5 "c5 : effective thermal capacity [J/(m²K)]"; c6 "c6 : wind dependence in the zero loss efficiency [s/m]"; tini "initial temperature [degree centigrade]"
      mask help: Model according to EN 12975 / ISO 22975
      mask Help: web(fullfile(path_carnot('help'),'Solar_Collector_basic.html'),'-helpbrowser')
      mask Display: disp('solar thermal\ncollector\nEN 12975')
  T_Ground_Undisturbed : Subsystem  mask(Undisturbed ground temperature){Tmeanoutside=0, deltathetae=10, tshift=0, cond_ground=1, rhocp=1000*2000, hh=10, znodes=10}
      mask prompts: Tmeanoutside "mean outside temperature over one year [°C]"; deltathetae "amplitude of monthly outside temperatures [°C]"; tshift "time shift where external temperature sine-curve shows a minimum [h]"; cond_ground "soil thermal conductivity in W/m/K"; rhocp "soil heat capacity per Volume in J/m³/K"; hh "depth z in m"; znodes "number of nodes"
      mask help:
      | The temperature of the undisturbed ground Tg is caclulated for a number of equidistant nodes from the surface down to a depth z.
      |
      | Tg = Tavg - dTavg * exp(-z/dg) * cos(2*pi*(t-ts)/t0 - z/dg) + G*z
      |
      | penetration depth : dg = sqrt(t0*cond/(pi*dens*cp))
      |
      | cond  : thermal conductivity of the ground in W/m/K
      | cp    : heat capacity of the ground in J/kg/K
      | dens  : density of the ground in kg/m³
      | G     : temperature increase in the depth (= 0.03 K/m)
      | t     : time of the year in seconds
      | t0    : total seconds of one year (= 3600*24*365)
      | ts    : time in seconds where the ambient temperature curve shows a minimum
      | Tavg  : annual mean ambient temperature
      | dTavg : annual amplitude of the ambient temperature
      | z     : depth in meters
      |
      | The equation is based on approaches presented in the literature for seasonal temperature variations in the earth’s crust (Baehr & Stephan 2006; Wesselak & Schabbach 2009), neglecting the influence of the heat transfer resistance from the ambient air to the surface of the ground (i.e. u_surf =):
      mask init:
      | %thermische eindringtiefe
      | delta_grd = sqrt((8760*3600*cond_ground)/(pi*rhocp));
      | 
      | % height vector
      | z = [0:hh/znodes:hh];
      mask Help: web(fullfile(path_carnot('help'),'T_Ground_Undisturbed.html'),'-helpbrowser')
      mask Display: plot(0,0,100,100,[90,10],[90,90],[50,50],[-0,90],[49,48,46,44,41,34,25,15],[-0,20,40,50,60,70,80,90],[52,54,56,58,61,67,76,85],[-0,20,40,50,60,70,80,90],[50,49,49,48,48,48,50,54,60],[-0,20,30,40,50,60,70,80,90],[50,51,51,52,52,50,48,43,35],[0,20,30,40,50,60,70,80,90])
  Thermal_Capacity : Subsystem  mask(Thermal Capacity){UA=1, mcp=4182*10, Tamb=20, cp_approx=4000}
      mask prompts: UA "Loss coefficient in W/K"; mcp "Thermal capacity in J/K"; Tamb "Ambient temperature in °C"; cp_approx "heat capacity of fluid in J/kg/K (approximate value)"
      mask help: Basic one node model of a thermal mass using the differential equation:
      mask Help: web(fullfile(path_carnot('help'),'Thermal_Capacity.html'),'-helpbrowser')
  Thermal_Node : Subsystem  mask(Thermal Capacity){UA=1, mcp=10*4182, cp_approx=4182, Tini=20}
      mask prompts: UA "Loss coefficient of node in W/K"; mcp "Thermal capacity of the node (mcp) in J/K"; cp_approx "Heat capacity of entering massflow in J/kg/K (approximate value)"; Tini "Initial temperature in °C"
      mask help:
      | Basic one node model of a thermal mass using the differential equation:
      | mcp * dT/dt = UA_loss*(Tamb-T) + mdot*cp_in*(Tin-T) + Qdot
      | Qdot: additional thermal power added to node
      | mdot: entering massflow
      | Tin: temperature of entering massflow
      mask Help: web(fullfile(path_carnot('help'),'Thermal_Capacity.html'),'-helpbrowser')
      mask Display: plot(-20,0,120,100,[10,70,70,10,10],[10,10,70,70,10],[70,90,90,30,10],[10,30,90,90,70],[90,70],[90,70],[50,30],[60,60],[40,40],[30,60])
  Wall_basic : Subsystem  mask(Wall basic){tau=tau, t0=t0, d=d, dactive=dactive, cond=cond, cwall=cwall, rho=rho}
      mask prompts: tau "Time constant in s"; t0 "Initial temperature in °C"; d "Thickness of layers in m"; dactive "Depth of active layer(s) in m"; cond "Conductivity of layer material in W/m/K"; cwall "Capacity of layer material in J/kg/K"; rho "Density of layer material in kg/m³"
      mask help: Basic model of a wall using a multilayer Beuken model.
      mask Help: web(fullfile(path_carnot('help'),'Wall_basic.html'),'-helpbrowser')
  sfun_storageTnodes : Subsystem  mask(S-Function Storage T-Nodes){dia=0.5, volume=0.5, standing=1, uloss=1.1, ubot=1.1, utop=1.1, cond=0.9, tini=20, nodes=10, nconnect=10}
      mask prompts: dia "diameter [m]"; volume "volume [m³]"; standing "standing cylinder"; uloss "heat transfer coefficient to ambient [W/m²K]"; ubot "heat transfer coefficient to ambient bottom [W/m²K]"; utop "heat transfer coefficient to ambient top [W/m²K]"; cond "effective thermal conductivity [W/mK]"; tini "initial temperature [°C]"; nodes "number of nodes [1]"; nconnect "number of ports [1]"
      mask help:
      | Basic 1xN Model for a storage tank based on the equation. The flow is calculated by the upwind scheme heat conduction between nodes by central differences (Patankar 1980).
      | (rho*cp) * dT/dt =U * Aloss / Vnode * (Tamb - Tnode)
      | + cond / dh2 * (Tnode_above - Tnode)
      | + cond / dh2 * (Tnode_below - Tnode)
      | + mdot_up * cp / Vnode * (Tnode_below - Tnode)
      | + mdot_down * cp / Vnode * (Tnode_above - Tnode)
      | + Uhx * Ahx / Vnode * (Thx_node - Tnode)
      mask init:
      | if (floor(nodes)-nodes>eps(nodes)) || nodes < 1.0
      |     error('The number of nodes must be a positve integer!');
      | end
      | 
      | if (floor(nconnect)-nconnect>eps(nconnect)) || nconnect < 1.0
      |     error('The number of ports must be a positve integer!');
      | end
      | 
      | 
      | 
      | if numel(tini)==1
      |     tini = ones(int32(nodes), 1)*tini;
      | else
      |     if numel(tini)~=int32(nodes)
      |         error('The initialisation temperature must be a scalar or a vector of size of number of nodes!');
      |     end
      | end
      | 
      | CarnotCallbacks_storage_Tnodes('InitCallback', gcb, nconnect);
      mask Help: web(fullfile(path_carnot('help'),'sfun_storageTnodes.html'),'-helpbrowser')
  sfun_storage_heatexchanger : Subsystem  mask(storage heat exchanger){idn=finned tube theoretical  - stratified, nodes=nodes, inlet=inlet, outlet=outlet, pp=[dpipe, swall, lpipe, cond, dfin, sfin, nfin]}
      mask prompts: idn "type"; nodes "number of nodes"; inlet "inlet node"; outlet "outlet node"; pp "parameter vector"
      mask init:
      | switch(idn)
      |     case 1
      |         id = 201;
      |     case 2
      |         id = 301;
      |     case 3
      |         id = 202;
      |     case 4
      |         id = 302;
      |     case 5
      |         id = 203;
      |     case 6
      |         id = 303;
      |     case 7
      |         id = 204;
      |     case 8
      |         id = 304;
      | end
      mask Help: web(['file:///' fullfile(path_carnot('help'),'StoragePorts_HeatExchangerModels.html')],'-helpbrowser')
      mask TypeOptions idn: smooth tube theoretical | smooth tube theoretical - stratified | finned tube theoretical | finned tube theoretical  - stratified | heat transfer from data fit | heat transfer from data fit  - stratified | heat transfer data fit EN12977 | heat transfer data fit EN12977  - stratified

== system carnot/Basic/Ventilation ==
  Window_Ventilation : Subsystem  mask(window ventilation){alpha=10, H=1, W=1}
      mask prompts: alpha "maximal opening angle (°)"; H "height of window (m)"; W "width of window (m)"
      mask help: Simulates the free driven ventilation through a window with an opening angle of [0,1]* max. angle. Valid for angles between 8° and 180°. Output is the VOLUME FLOW RATE in m^3/s. Calculation based on the Ansatz from Weber.
      mask Display: plot(0,10,90,80,[20 70 70 20 20],[20 20 70 70 20],[20 70 80 30 20],[20 20 65 65 20])
